simulink model "two_balloons_empirical"  (R2020b)
settings: Solver=VariableStepAuto  StartTime=0.0  StopTime=60*5  FixedStep=0.001  RelTol=1e-3
InitFcn:
  | seed1 = randi(100000);
  | seed2 = randi(200000);
model workspace (MAT data in the model file):
  dCoupling = 10
  kCoupling = 10
values from neighbouring files (symbols this model uses):
  bm = 2/1000    (= 0.002)    [optimiseB2.m]    (also in optimiseBO.m)
  Cd = a(4)    [comparisonPlot.m]    (also in optimiseB2.m = 0.185; optimiseBO.m = 0.185; params2.m = 0.185; sim_2balloon.m = 0.185)
  nH = x2nn.nH    [optimiseB2.m]    (also in optimiseBO.m = x.nH; params2.m = 10; sim_2balloon.m = x(2); sim_balloon.m = x(2))
  normalScaling = x2ll.normalScaling    [optimiseB2.m]    (also in optimiseBO.m = x.normalScaling; params2.m = 1; sim_2balloon.m = 0.259830816053; sim_balloon.m = x(5))
  nS = 1    [comparisonPlot.m]    (also in optimiseB2.m = x2nn.nS; optimiseBO.m = x.nS; params2.m = 0.025; sim_2balloon.m = x(3))
  nV = a(7)    [comparisonPlot.m]    (also in optimiseB2.m = x2nn.nV; optimiseBO.m = x.nV; params2.m = 0.5; sim_2balloon.m = x(1))
  rb = 0.16    [comparisonPlot.m]    (also in optimiseB2.m = 0.08; optimiseBO.m = 0.08; params2.m = 0.08; sim_2balloon.m = 0.08)
  rn = a(1)    [comparisonPlot.m]    (also in optimiseB2.m = 0.0625; optimiseBO.m = 0.0625; params2.m = 0.0625; sim_2balloon.m = 0.0625)
  seedX = randi(100000)    [optimiseB2.m]    (also in optimiseBO.m; params2.m; sim_2balloon.m; sim_balloon.m)
  seedX1 = randi(100000)    [optimiseB2.m]    (also in params2.m; sim_2balloon.m)
  seedY = randi(100000)    [optimiseB2.m]    (also in optimiseBO.m; params2.m; sim_2balloon.m; sim_balloon.m)
  seedY1 = randi(100000)    [optimiseB2.m]    (also in params2.m; sim_2balloon.m)
  seedZ = randi(100000)    [optimiseB2.m]    (also in optimiseBO.m; params2.m; sim_2balloon.m; sim_balloon.m)
  seedZ1 = randi(100000)    [optimiseB2.m]    (also in params2.m; sim_2balloon.m)
  theta = a(2)    [comparisonPlot.m]    (also in extract3D.m = deg2rad(-5); optimiseB2.m = x2ll.theta; optimiseBO.m = x.theta; params2.m = 3.5)
  V0 = a(3)    [comparisonPlot.m]    (also in optimiseB2.m = x2ll.V0; optimiseBO.m = x.V0; params2.m = 3.7; sim_2balloon.m = 1.01295922371)
undefined symbols (not defined in the file or in its folder): bm1
libraries: nesl_utility x19, sm_lib x10, eeGeneralControl x6
settings Model: Creator=toby  LastModifiedBy=BIRL

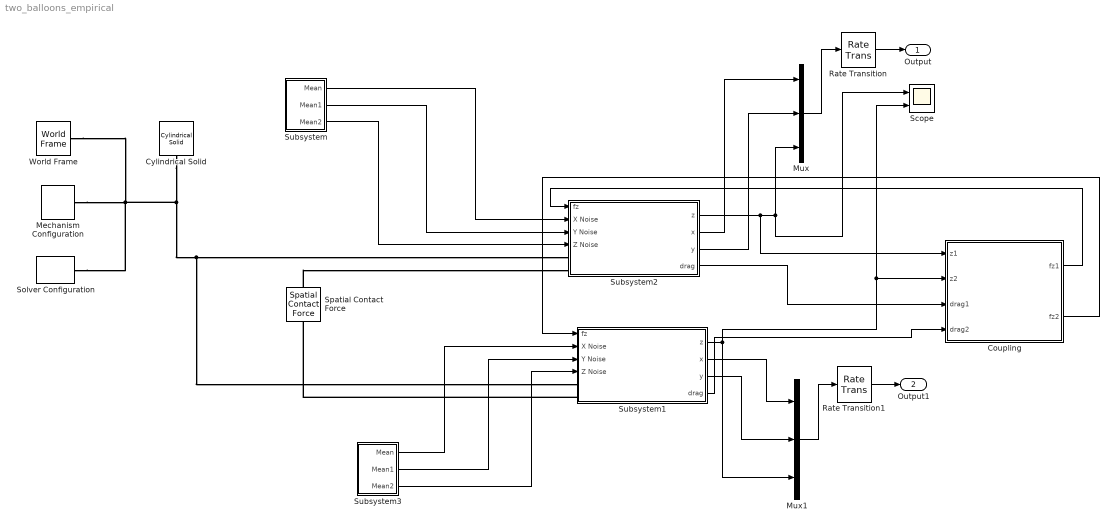
== system two_balloons_empirical ==
  Coupling : Subsystem
  Cylindrical Solid : sm_lib/Body Elements/Cylindrical Solid  GraphicAmbientColor=[0.15 0.15 0.15 1.0]  BasedOnType=Density  CenterOfMass=[0 0 0]  CenterOfMassUnits=m  GraphicDiffuseColor=[1.0 1.0 0.0]  CylinderLength=0.01  CylinderLengthUnits=m  CylinderRadius=rn  CylinderRadiusUnits=m  Density=1000  DensityUnits=kg/m^3  DoExposeReferenceFrame=on  GraphicEmissiveColor=[0.0 0.0 0.0 1.0]  ExportEntireGeometry=off  SerializedFrames=<Frames/>  MarkerShape=Sphere  MarkerSize=10  GraphicType=FromGeometry  InertiaType=CalculateFromGeometry  Mass=1  MassUnits=kg  MomentsOfInertia=[1 1 1]  MomentsOfInertiaUnits=kg*m^2  GraphicOpacity=1.0  ProductsOfInertia=[0 0 0]  ProductsOfInertiaUnits=kg*m^2  GraphicShininess=75  GraphicSpecularColor=[0.5 0.5 0.5 1.0]  GraphicVisPropType=SimpleVisualProperties
  Mechanism Configuration : sm_lib/Utilities/Mechanism Configuration  UniformGravity=Constant  GravityVector=[0 0 -9.81]  GravityVectorUnits=m/s^2  GravityUnits=m/s^2  LinearizationDelta=0.001  JointModeTransitionNonlinearIterations=2
  Mux : Mux  Inputs=3
  Mux1 : Mux  Inputs=3
  Rate Transition : RateTransition  OutPortSampleTime=1/40
  Rate Transition1 : RateTransition  OutPortSampleTime=1/40
  Scope : Scope  NumInputPorts=2
  Solver Configuration : nesl_utility/Solver Configuration  PhysicalDomain=network_engine_domain  SubClassName=solver  LeftPortType=input  RightPortType=generic  Tones=[]  Harmonics=[]  SimulateNoise=off  Profile=off  UseLocalSampling=off  EnableSwitchedLinearOptims=on  FrequencyDomain=off  UseCCode=off  RelTol=0.001  AbsTol=1e-06  MinStep=1e-09  ToWorkspace=off  RevertToSquareIcSolve=off  NumHomotopyIterations=100  PhasorMode=off  PhasorModeNumHarmonics=1  DoDC=off  ResidualTolerance=1e-9  UseLocalSolver=off  LocalSolverChoice=NE_BACKWARD_EULER_ADVANCER  LocalSolverSampleTime=.001  DoFixedCost=off  MaxNonlinIter=3  MaxModeIter=2  ComputeImpulses=off  ImpulseIterations=2  LinearAlgebra=Sparse  EquationFormulation=NE_TIME_EF  DelaysMemoryBudget=1024  AutomaticFiltering=on  FilteringTimeConstant=0.001  PartitionStorageMethod=AS_NEEDED  PartitionMemoryBudget=1024  PartitionMethod=FAST
  Spatial Contact Force : sm_lib/Forces and Torques/Spatial Contact Force  CoefficientOfDynamicFriction=0.1  CoefficientOfStaticFriction=0.1  NormalDamping=d  NormalDampingUnits=N/(m/s)  NormalStiffness=k  NormalStiffnessUnits=N/m  FrictionalCriticalVelocity=1e-3  FrictionalCriticalVelocityUnits=m/s  ZeroCrossDetectContactStartAndEnd=off  SenseFrictionalForceMagnitude=off  SenseNormalForceMagnitude=off  SenseSeparationDistance=off  NormalTransitionRegionWidth=tw  NormalTransitionRegionWidthUnits=m  FrictionType=SmoothStickSlip
  Subsystem : Subsystem
  Subsystem1 : Subsystem  mask{initialHeight=0.5, ix=0, iy=0, balloonRadius=80/1000, balloonMass=bm1}
      mask prompts: initialHeight "initial height"; balloonRadius "balloon radius"; balloonMass "balloon mass"
  Subsystem2 : Subsystem  mask{initialHeight=0.2, ix=0, iy=0, balloonRadius=80/1000, balloonMass=bm}
      mask prompts: initialHeight "initial height"; balloonRadius "balloon radius"; balloonMass "balloon mass"
  Subsystem3 : Subsystem
  World Frame : sm_lib/Frames and Transforms/World Frame
  Output : Outport
  Output1 : Outport  Port=2
  wires:
  Subsystem2/1(z) -> Coupling/1(z1), Scope/1, Mux/3
  Subsystem2/2(x) -> Mux/1
  Subsystem1/1(z) -> Scope/2, Coupling/2(z2), Mux1/3
  Subsystem1/2(x) -> Mux1/1
  Subsystem2/3(y) -> Mux/2
  Subsystem1/3(y) -> Mux1/2
  Rate Transition/1 -> Output/1
  Mux/1 -> Rate Transition/1
  Rate Transition1/1 -> Output1/1
  Mux1/1 -> Rate Transition1/1
  Coupling/1(fz1) -> Subsystem2/1(fz)
  Coupling/2(fz2) -> Subsystem1/1(fz)
  Subsystem2/4(drag) -> Coupling/3(drag1)
  Subsystem1/4(drag) -> Coupling/4(drag2)
  Subsystem/1(" Mean") -> Subsystem2/2(X Noise)
  Subsystem/2(" Mean1") -> Subsystem2/3(Y Noise)
  Subsystem/3(" Mean2") -> Subsystem2/4(Z Noise)
  Subsystem3/1(" Mean") -> Subsystem1/2(X Noise)
  Subsystem3/2(" Mean1") -> Subsystem1/3(Y Noise)
  Subsystem3/3(" Mean2") -> Subsystem1/4(Z Noise)
  connections:
  Solver Configuration/RConn1 -- Cylindrical Solid/RConn1 -- Subsystem1/LConn1 -- Subsystem2/LConn1 -- World Frame/RConn1 -- Mechanism Configuration/RConn1
  Spatial Contact Force/LConn1 -- Subsystem2/LConn2
  Subsystem1/LConn2 -- Spatial Contact Force/RConn1

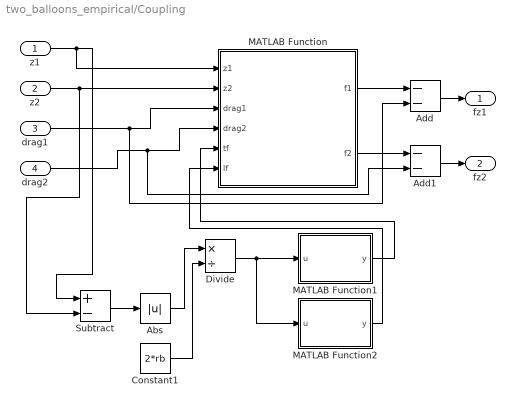
== system two_balloons_empirical/Coupling ==
  z1 : Inport
  z2 : Inport  Port=2
  drag1 : Inport  Port=3
  drag2 : Inport  Port=4
  Abs : Abs
  Add : Sum  Inputs=--
  Add1 : Sum  Inputs=--
  Constant1 : Constant  Value=2*rb
  Divide : Product  Inputs=*/
  MATLAB Function : MATLAB Function  TreatAsAtomicUnit=on
  MATLAB Function1 : MATLAB Function  TreatAsAtomicUnit=on
  MATLAB Function2 : MATLAB Function  TreatAsAtomicUnit=on
  Subtract : Sum  Inputs=+-
  fz1 : Outport
  fz2 : Outport  Port=2
  wires:
  drag1/1 -> Add/2, MATLAB Function/3(drag1)
  drag2/1 -> Add1/2, MATLAB Function/4(drag2)
  z1/1 -> MATLAB Function/1(z1), Subtract/1
  z2/1 -> Subtract/2, MATLAB Function/2(z2)
  Subtract/1 -> Abs/1
  Abs/1 -> Divide/1
  Constant1/1 -> Divide/2
  Divide/1 -> MATLAB Function2/1(u), MATLAB Function1/1(u)
  MATLAB Function1/1(y) -> MATLAB Function/5(tf)
  MATLAB Function2/1(y) -> MATLAB Function/6(lf)
  Add1/1 -> fz2/1
  Add/1 -> fz1/1
  MATLAB Function/1(f1) -> Add/1
  MATLAB Function/2(f2) -> Add1/1

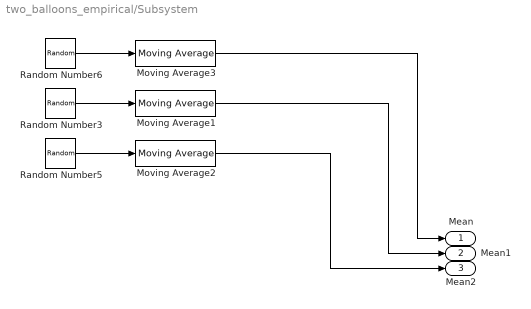
== system two_balloons_empirical/Subsystem ==
  Moving Average1 : eeGeneralControl/Moving Average  VariantControl=Variant1  LabelModeActiveChoice=Discrete  f=10  x0=0  Ts=nS/10
      settings: SourceProductBaseCode=PS
  Moving Average2 : eeGeneralControl/Moving Average  VariantControl=Variant1  LabelModeActiveChoice=Discrete  f=10  x0=0  Ts=nS/10
      settings: SourceProductBaseCode=PS
  Moving Average3 : eeGeneralControl/Moving Average  VariantControl=Variant1  LabelModeActiveChoice=Discrete  f=10  x0=0  Ts=nS/10
      settings: SourceProductBaseCode=PS
  Random Number3 : RandomNumber  Variance=nH  Seed=seedY  SampleTime=nS
  Random Number5 : RandomNumber  Variance=nV  Seed=seedZ  SampleTime=nS
  Random Number6 : RandomNumber  Variance=nH  Seed=seedX  SampleTime=nS
  " Mean" : Outport
  " Mean1" : Outport  Port=2
  " Mean2" : Outport  Port=3
  wires:
  Random Number3/1 -> Moving Average1/1
  Random Number5/1 -> Moving Average2/1
  Random Number6/1 -> Moving Average3/1
  Moving Average3/1 -> " Mean"/1
  Moving Average1/1 -> " Mean1"/1
  Moving Average2/1 -> " Mean2"/1

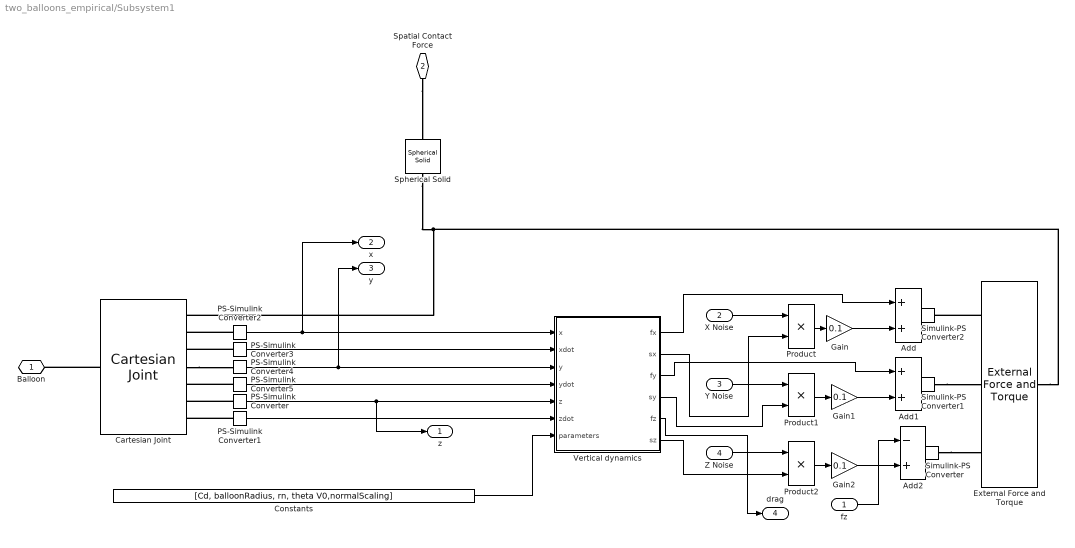
== system two_balloons_empirical/Subsystem1 ==
  fz : Inport
  X Noise : Inport  Port=2
  Y Noise : Inport  Port=3
  Z Noise : Inport  Port=4
  Add : Sum
  Add1 : Sum
  Add2 : Sum  Inputs=-+
  Cartesian Joint : sm_lib/Joints/Cartesian Joint  JointMode=Normal  SenseConstraintForce=off  SenseConstraintForceX=off  SenseConstraintForceY=off  SenseConstraintForceZ=off  SenseConstraintTorque=off  SenseConstraintTorqueX=off  SenseConstraintTorqueY=off  SenseConstraintTorqueZ=off  SenseTotalForce=off  SenseTotalForceX=off  SenseTotalForceY=off  SenseTotalForceZ=off  SenseTotalTorque=off  SenseTotalTorqueX=off  SenseTotalTorqueY=off  SenseTotalTorqueZ=off  CompositeWrenchDir=FollowerOnBase  CompositeWrenchFrame=BaseFrame  PxEquilibriumPosition=0  PxEquilibriumPositionUnits=m  PxSpringStiffness=0  PxSpringStiffnessUnits=N/m  PxDampingCoefficient=hd  PxDampingCoefficientUnits=N/(m/s)  PxTorqueActuationMode=NoTorque  PxMotionActuationMode=ComputedMotion  PxSensePosition=on  PxSenseVelocity=on  PxSenseAcceleration=off  PxSenseTorqueForce=off  PxSenseLowerLimitTorqueForce=off  PxSenseUpperLimitTorqueForce=off  PxLowerLimitSpecify=on  PxLowerLimitBound=-0.1  PxLowerLimitBoundUnits=m  PxLowerLimitStiffness=1e6  PxLowerLimitStiffnessUnits=N/m  PxLowerLimitDamping=1e3  PxLowerLimitDampingUnits=N/(m/s)  PxLowerLimitTransitionRegionWidth=1e-4  PxLowerLimitTransitionRegionWidthUnits=m  PxUpperLimitSpecify=on  PxUpperLimitBound=0.1  PxUpperLimitBoundUnits=m  PxUpperLimitStiffness=1e6  PxUpperLimitStiffnessUnits=N/m  PxUpperLimitDamping=1e3  PxUpperLimitDampingUnits=N/(m/s)  PxUpperLimitTransitionRegionWidth=1e-4  PxUpperLimitTransitionRegionWidthUnits=m  PxPositionTargetSpecify=on  PxPositionTargetPriority=High  PxPositionTargetValue=ix  PxPositionTargetValueUnits=m  PxVelocityTargetSpecify=off  PxVelocityTargetPriority=High  PxVelocityTargetValue=-0.75  PxVelocityTargetValueUnits=m/s  PyEquilibriumPosition=0  PyEquilibriumPositionUnits=m  PySpringStiffness=0  PySpringStiffnessUnits=N/m  PyDampingCoefficient=hd  PyDampingCoefficientUnits=N/(m/s)  PyTorqueActuationMode=NoTorque  PyMotionActuationMode=ComputedMotion  PySensePosition=on  PySenseVelocity=on  PySenseAcceleration=off  PySenseTorqueForce=off  PySenseLowerLimitTorqueForce=off  PySenseUpperLimitTorqueForce=off  PyLowerLimitSpecify=on  PyLowerLimitBound=-0.1  PyLowerLimitBoundUnits=m  PyLowerLimitStiffness=1e6  PyLowerLimitStiffnessUnits=N/m  PyLowerLimitDamping=1e3  PyLowerLimitDampingUnits=N/(m/s)  PyLowerLimitTransitionRegionWidth=1e-4  PyLowerLimitTransitionRegionWidthUnits=m  PyUpperLimitSpecify=on  PyUpperLimitBound=0.1  PyUpperLimitBoundUnits=m  PyUpperLimitStiffness=1e6  PyUpperLimitStiffnessUnits=N/m  PyUpperLimitDamping=1e3  PyUpperLimitDampingUnits=N/(m/s)  PyUpperLimitTransitionRegionWidth=1e-4  PyUpperLimitTransitionRegionWidthUnits=m  PyPositionTargetSpecify=on  PyPositionTargetPriority=High  PyPositionTargetValue=iy  PyPositionTargetValueUnits=m  PyVelocityTargetSpecify=off  PyVelocityTargetPriority=High  PyVelocityTargetValue=0  PyVelocityTargetValueUnits=m/s  PzEquilibriumPosition=0  PzEquilibriumPositionUnits=m  PzSpringStiffness=0  PzSpringStiffnessUnits=N/m  PzDampingCoefficient=0  PzDampingCoefficientUnits=N/(m/s)  PzTorqueActuationMode=NoTorque  PzMotionActuationMode=ComputedMotion  PzSensePosition=on  PzSenseVelocity=on  PzSenseAcceleration=off  PzSenseTorqueForce=off  PzSenseLowerLimitTorqueForce=off  PzSenseUpperLimitTorqueForce=off  PzLowerLimitSpecify=on  PzLowerLimitBound=0.1  PzLowerLimitBoundUnits=m  PzLowerLimitStiffness=1e6  PzLowerLimitStiffnessUnits=N/m  PzLowerLimitDamping=1e3  PzLowerLimitDampingUnits=N/(m/s)  PzLowerLimitTransitionRegionWidth=1e-4  PzLowerLimitTransitionRegionWidthUnits=m  PzUpperLimitSpecify=on  PzUpperLimitBound=1.7  PzUpperLimitBoundUnits=m  PzUpperLimitStiffness=1e6  PzUpperLimitStiffnessUnits=N/m  PzUpperLimitDamping=1e3  PzUpperLimitDampingUnits=N/(m/s)  PzUpperLimitTransitionRegionWidth=1e-4  PzUpperLimitTransitionRegionWidthUnits=m  PzPositionTargetSpecify=on  PzPositionTargetPriority=High  PzPositionTargetValue=initialHeight  PzPositionTargetValueUnits=m  PzVelocityTargetSpecify=off  PzVelocityTargetPriority=High  PzVelocityTargetValue=2.5  PzVelocityTargetValueUnits=m/s
  Constants : Constant  Value=[Cd, balloonRadius, rn, theta V0,normalScaling]
  External Force and Torque : sm_lib/Forces and Torques/External Force and Torque  ForceResolutionFrame=AttachedFrame  EnableForceX=on  EnableForceY=on  EnableForceZ=on  EnableForce=off  TorqueResolutionFrame=AttachedFrame  EnableTorqueX=off  EnableTorqueY=off  EnableTorqueZ=off  EnableTorque=off
  Gain : Gain  Gain=0.1
  Gain1 : Gain  Gain=0.1
  Gain2 : Gain  Gain=0.1
  PS-Simulink Converter{,1..5} (6 alike) : nesl_utility/PS-Simulink Converter  PhysicalDomain=network_engine_domain  SubClassName=ps_output  LeftPortType=input  RightPortType=output  PseudoPeriodic=off  Frequencies=[]  Unit=inherit  AffineConversion=off
  Product : Product
  Product1 : Product
  Product2 : Product
  Simulink-PS Converter : nesl_utility/Simulink-PS Converter  PhysicalDomain=network_engine_domain  SubClassName=ps_input  LeftPortType=input  RightPortType=output  PseudoPeriodic=off  Frequencies=[]  NoiseDistribution=none  NoiseParameters=[]  Unit=1  AffineConversion=off  FilteringAndDerivatives=provide  SimscapeFilterOrder=1  InputFilterTimeConstant=0.001  UdotUserProvided=0
  Simulink-PS Converter1 : nesl_utility/Simulink-PS Converter  PhysicalDomain=network_engine_domain  SubClassName=ps_input  LeftPortType=input  RightPortType=output  PseudoPeriodic=off  Frequencies=[]  NoiseDistribution=none  NoiseParameters=[]  Unit=1  AffineConversion=off  FilteringAndDerivatives=provide  SimscapeFilterOrder=1  InputFilterTimeConstant=0.001  UdotUserProvided=0
  Simulink-PS Converter2 : nesl_utility/Simulink-PS Converter  PhysicalDomain=network_engine_domain  SubClassName=ps_input  LeftPortType=input  RightPortType=output  PseudoPeriodic=off  Frequencies=[]  NoiseDistribution=none  NoiseParameters=[]  Unit=1  AffineConversion=off  FilteringAndDerivatives=provide  SimscapeFilterOrder=1  InputFilterTimeConstant=0.001  UdotUserProvided=0
  Spherical Solid : sm_lib/Body Elements/Spherical Solid  GraphicAmbientColor=[0.15 0.15 0.15 1.0]  BasedOnType=Mass  CenterOfMass=[0 0 0]  CenterOfMassUnits=m  GraphicDiffuseColor=[1.0 0.0 0.2]  Density=1000  DensityUnits=kg/m^3  DoExposeReferenceFrame=on  GraphicEmissiveColor=[0.0 0.0 0.0 1.0]  ExportEntireGeometry=on  SerializedExposedGeometries=<ExposedGeometries><ExposedGeometry><RawGeometryId>entire</RawGeometryId><ExposedGeometryId>G</ExposedGeometryId></ExposedGeometry></ExposedGeometries>  SerializedFrames=<Frames/>  MarkerShape=Sphere  MarkerSize=10  GraphicType=FromGeometry  InertiaType=CalculateFromGeometry  Mass=balloonMass  MassUnits=kg  MomentsOfInertia=[1 1 1]  MomentsOfInertiaUnits=kg*m^2  GraphicOpacity=1.0  ProductsOfInertia=[0 0 0]  ProductsOfInertiaUnits=kg*m^2  GraphicShininess=75  GraphicSpecularColor=[0.5 0.5 0.5 1.0]  SphereRadius=balloonRadius  SphereRadiusUnits=m  GraphicVisPropType=SimpleVisualProperties
  Vertical dynamics : MATLAB Function  TreatAsAtomicUnit=on
  Balloon : PMIOPort  Side=Left
  Spatial Contact Force : PMIOPort  Port=2  Side=Left
  z : Outport
  x : Outport  Port=2
  y : Outport  Port=3
  drag : Outport  Port=4
  wires:
  PS-Simulink Converter3/1 -> Vertical dynamics/2(xdot)
  PS-Simulink Converter5/1 -> Vertical dynamics/4(ydot)
  Constants/1 -> Vertical dynamics/7(parameters)
  PS-Simulink Converter1/1 -> Vertical dynamics/6(zdot)
  Vertical dynamics/6(sz) -> Product2/2
  X Noise/1 -> Product/1
  Vertical dynamics/4(sy) -> Product1/2
  Z Noise/1 -> Product2/1
  Y Noise/1 -> Product1/1
  Vertical dynamics/2(sx) -> Product/2
  Vertical dynamics/5(fz) -> drag/1
  Vertical dynamics/1(fx) -> Add/1
  Vertical dynamics/3(fy) -> Add1/1
  Add1/1 -> Simulink-PS Converter1/1
  Add/1 -> Simulink-PS Converter2/1
  Product/1 -> Gain/1
  Gain/1 -> Add/2
  Product1/1 -> Gain1/1
  Gain1/1 -> Add1/2
  Product2/1 -> Gain2/1
  Gain2/1 -> Add2/2
  Add2/1 -> Simulink-PS Converter/1
  fz/1 -> Add2/1
  PS-Simulink Converter2/1 -> Vertical dynamics/1(x), x/1
  PS-Simulink Converter4/1 -> Vertical dynamics/3(y), y/1
  PS-Simulink Converter/1 -> Vertical dynamics/5(z), z/1
  connections:
  PS-Simulink Converter/LConn1 -- Cartesian Joint/RConn6
  PS-Simulink Converter2/LConn1 -- Cartesian Joint/RConn2
  Spherical Solid/RConn1 -- External Force and Torque/RConn1 -- Cartesian Joint/RConn1
  Cartesian Joint/LConn1 -- Balloon/RConn1
  PS-Simulink Converter5/LConn1 -- Cartesian Joint/RConn5
  Cartesian Joint/RConn4 -- PS-Simulink Converter4/LConn1
  PS-Simulink Converter3/LConn1 -- Cartesian Joint/RConn3
  PS-Simulink Converter1/LConn1 -- Cartesian Joint/RConn7
  Spatial Contact Force/RConn1 -- Spherical Solid/LConn1
  External Force and Torque/LConn1 -- Simulink-PS Converter2/RConn1
  Simulink-PS Converter1/RConn1 -- External Force and Torque/LConn2
  Simulink-PS Converter/RConn1 -- External Force and Torque/LConn3

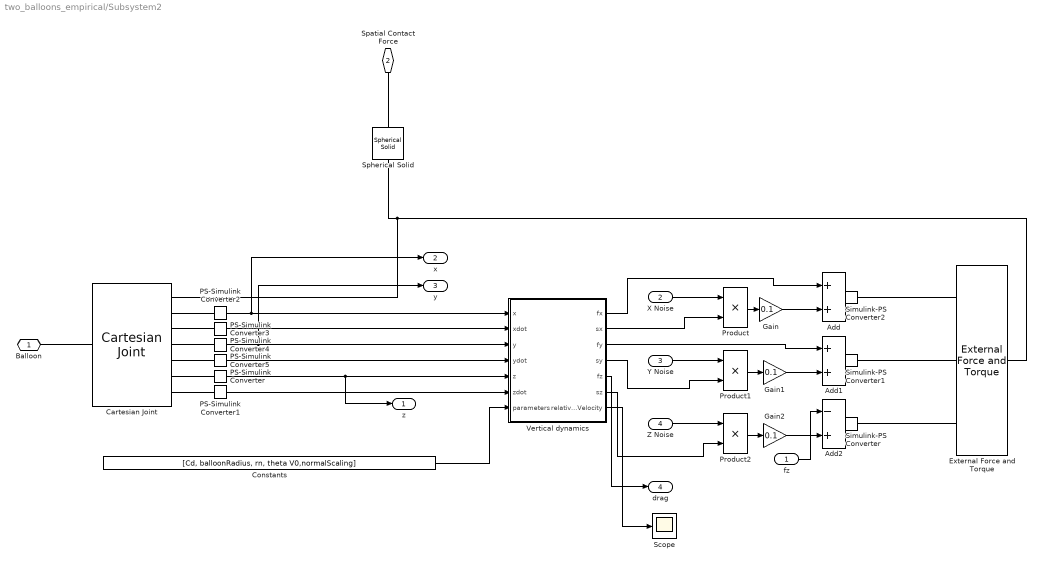
== system two_balloons_empirical/Subsystem2 ==
  fz : Inport
  X Noise : Inport  Port=2
  Y Noise : Inport  Port=3
  Z Noise : Inport  Port=4
  Add : Sum
  Add1 : Sum
  Add2 : Sum  Inputs=-+
  Cartesian Joint : sm_lib/Joints/Cartesian Joint  JointMode=Normal  SenseConstraintForce=off  SenseConstraintForceX=off  SenseConstraintForceY=off  SenseConstraintForceZ=off  SenseConstraintTorque=off  SenseConstraintTorqueX=off  SenseConstraintTorqueY=off  SenseConstraintTorqueZ=off  SenseTotalForce=off  SenseTotalForceX=off  SenseTotalForceY=off  SenseTotalForceZ=off  SenseTotalTorque=off  SenseTotalTorqueX=off  SenseTotalTorqueY=off  SenseTotalTorqueZ=off  CompositeWrenchDir=FollowerOnBase  CompositeWrenchFrame=BaseFrame  PxEquilibriumPosition=0  PxEquilibriumPositionUnits=m  PxSpringStiffness=0  PxSpringStiffnessUnits=N/m  PxDampingCoefficient=hd  PxDampingCoefficientUnits=N/(m/s)  PxTorqueActuationMode=NoTorque  PxMotionActuationMode=ComputedMotion  PxSensePosition=on  PxSenseVelocity=on  PxSenseAcceleration=off  PxSenseTorqueForce=off  PxSenseLowerLimitTorqueForce=off  PxSenseUpperLimitTorqueForce=off  PxLowerLimitSpecify=on  PxLowerLimitBound=-0.1  PxLowerLimitBoundUnits=m  PxLowerLimitStiffness=1e6  PxLowerLimitStiffnessUnits=N/m  PxLowerLimitDamping=1e3  PxLowerLimitDampingUnits=N/(m/s)  PxLowerLimitTransitionRegionWidth=1e-4  PxLowerLimitTransitionRegionWidthUnits=m  PxUpperLimitSpecify=on  PxUpperLimitBound=0.1  PxUpperLimitBoundUnits=m  PxUpperLimitStiffness=1e6  PxUpperLimitStiffnessUnits=N/m  PxUpperLimitDamping=1e3  PxUpperLimitDampingUnits=N/(m/s)  PxUpperLimitTransitionRegionWidth=1e-4  PxUpperLimitTransitionRegionWidthUnits=m  PxPositionTargetSpecify=on  PxPositionTargetPriority=High  PxPositionTargetValue=ix  PxPositionTargetValueUnits=m  PxVelocityTargetSpecify=off  PxVelocityTargetPriority=High  PxVelocityTargetValue=-0.75  PxVelocityTargetValueUnits=m/s  PyEquilibriumPosition=0  PyEquilibriumPositionUnits=m  PySpringStiffness=0  PySpringStiffnessUnits=N/m  PyDampingCoefficient=hd  PyDampingCoefficientUnits=N/(m/s)  PyTorqueActuationMode=NoTorque  PyMotionActuationMode=ComputedMotion  PySensePosition=on  PySenseVelocity=on  PySenseAcceleration=off  PySenseTorqueForce=off  PySenseLowerLimitTorqueForce=off  PySenseUpperLimitTorqueForce=off  PyLowerLimitSpecify=on  PyLowerLimitBound=-0.1  PyLowerLimitBoundUnits=m  PyLowerLimitStiffness=1e6  PyLowerLimitStiffnessUnits=N/m  PyLowerLimitDamping=1e3  PyLowerLimitDampingUnits=N/(m/s)  PyLowerLimitTransitionRegionWidth=1e-4  PyLowerLimitTransitionRegionWidthUnits=m  PyUpperLimitSpecify=on  PyUpperLimitBound=0.1  PyUpperLimitBoundUnits=m  PyUpperLimitStiffness=1e6  PyUpperLimitStiffnessUnits=N/m  PyUpperLimitDamping=1e3  PyUpperLimitDampingUnits=N/(m/s)  PyUpperLimitTransitionRegionWidth=1e-4  PyUpperLimitTransitionRegionWidthUnits=m  PyPositionTargetSpecify=on  PyPositionTargetPriority=High  PyPositionTargetValue=iy  PyPositionTargetValueUnits=m  PyVelocityTargetSpecify=off  PyVelocityTargetPriority=High  PyVelocityTargetValue=0  PyVelocityTargetValueUnits=m/s  PzEquilibriumPosition=0  PzEquilibriumPositionUnits=m  PzSpringStiffness=0  PzSpringStiffnessUnits=N/m  PzDampingCoefficient=0  PzDampingCoefficientUnits=N/(m/s)  PzTorqueActuationMode=NoTorque  PzMotionActuationMode=ComputedMotion  PzSensePosition=on  PzSenseVelocity=on  PzSenseAcceleration=off  PzSenseTorqueForce=off  PzSenseLowerLimitTorqueForce=off  PzSenseUpperLimitTorqueForce=off  PzLowerLimitSpecify=on  PzLowerLimitBound=0.1  PzLowerLimitBoundUnits=m  PzLowerLimitStiffness=1e6  PzLowerLimitStiffnessUnits=N/m  PzLowerLimitDamping=1e3  PzLowerLimitDampingUnits=N/(m/s)  PzLowerLimitTransitionRegionWidth=1e-4  PzLowerLimitTransitionRegionWidthUnits=m  PzUpperLimitSpecify=on  PzUpperLimitBound=1.7  PzUpperLimitBoundUnits=m  PzUpperLimitStiffness=1e6  PzUpperLimitStiffnessUnits=N/m  PzUpperLimitDamping=1e3  PzUpperLimitDampingUnits=N/(m/s)  PzUpperLimitTransitionRegionWidth=1e-4  PzUpperLimitTransitionRegionWidthUnits=m  PzPositionTargetSpecify=on  PzPositionTargetPriority=High  PzPositionTargetValue=initialHeight  PzPositionTargetValueUnits=m  PzVelocityTargetSpecify=off  PzVelocityTargetPriority=High  PzVelocityTargetValue=2.5  PzVelocityTargetValueUnits=m/s
  Constants : Constant  Value=[Cd, balloonRadius, rn, theta V0,normalScaling]
  External Force and Torque : sm_lib/Forces and Torques/External Force and Torque  ForceResolutionFrame=AttachedFrame  EnableForceX=on  EnableForceY=on  EnableForceZ=on  EnableForce=off  TorqueResolutionFrame=AttachedFrame  EnableTorqueX=off  EnableTorqueY=off  EnableTorqueZ=off  EnableTorque=off
  Gain : Gain  Gain=0.1
  Gain1 : Gain  Gain=0.1
  Gain2 : Gain  Gain=0.1
  PS-Simulink Converter{,1..5} (6 alike) : nesl_utility/PS-Simulink Converter  PhysicalDomain=network_engine_domain  SubClassName=ps_output  LeftPortType=input  RightPortType=output  PseudoPeriodic=off  Frequencies=[]  Unit=inherit  AffineConversion=off
  Product : Product
  Product1 : Product
  Product2 : Product
  Scope : Scope
  Simulink-PS Converter : nesl_utility/Simulink-PS Converter  PhysicalDomain=network_engine_domain  SubClassName=ps_input  LeftPortType=input  RightPortType=output  PseudoPeriodic=off  Frequencies=[]  NoiseDistribution=none  NoiseParameters=[]  Unit=1  AffineConversion=off  FilteringAndDerivatives=provide  SimscapeFilterOrder=1  InputFilterTimeConstant=0.001  UdotUserProvided=0
  Simulink-PS Converter1 : nesl_utility/Simulink-PS Converter  PhysicalDomain=network_engine_domain  SubClassName=ps_input  LeftPortType=input  RightPortType=output  PseudoPeriodic=off  Frequencies=[]  NoiseDistribution=none  NoiseParameters=[]  Unit=1  AffineConversion=off  FilteringAndDerivatives=provide  SimscapeFilterOrder=1  InputFilterTimeConstant=0.001  UdotUserProvided=0
  Simulink-PS Converter2 : nesl_utility/Simulink-PS Converter  PhysicalDomain=network_engine_domain  SubClassName=ps_input  LeftPortType=input  RightPortType=output  PseudoPeriodic=off  Frequencies=[]  NoiseDistribution=none  NoiseParameters=[]  Unit=1  AffineConversion=off  FilteringAndDerivatives=provide  SimscapeFilterOrder=1  InputFilterTimeConstant=0.001  UdotUserProvided=0
  Spherical Solid : sm_lib/Body Elements/Spherical Solid  GraphicAmbientColor=[0.15 0.15 0.15 1.0]  BasedOnType=Mass  CenterOfMass=[0 0 0]  CenterOfMassUnits=m  GraphicDiffuseColor=[0.0 0.0 1.0]  Density=1000  DensityUnits=kg/m^3  DoExposeReferenceFrame=on  GraphicEmissiveColor=[0.0 0.0 0.0 1.0]  ExportEntireGeometry=on  SerializedExposedGeometries=<ExposedGeometries><ExposedGeometry><RawGeometryId>entire</RawGeometryId><ExposedGeometryId>G</ExposedGeometryId></ExposedGeometry></ExposedGeometries>  SerializedFrames=<Frames/>  MarkerShape=Sphere  MarkerSize=10  GraphicType=FromGeometry  InertiaType=CalculateFromGeometry  Mass=balloonMass  MassUnits=kg  MomentsOfInertia=[1 1 1]  MomentsOfInertiaUnits=kg*m^2  GraphicOpacity=1.0  ProductsOfInertia=[0 0 0]  ProductsOfInertiaUnits=kg*m^2  GraphicShininess=75  GraphicSpecularColor=[0.5 0.5 0.5 1.0]  SphereRadius=balloonRadius  SphereRadiusUnits=m  GraphicVisPropType=SimpleVisualProperties
  Vertical dynamics : MATLAB Function  TreatAsAtomicUnit=on
  Balloon : PMIOPort  Side=Left
  Spatial Contact Force : PMIOPort  Port=2  Side=Left
  z : Outport
  x : Outport  Port=2
  y : Outport  Port=3
  drag : Outport  Port=4
  wires:
  PS-Simulink Converter3/1 -> Vertical dynamics/2(xdot)
  PS-Simulink Converter5/1 -> Vertical dynamics/4(ydot)
  Constants/1 -> Vertical dynamics/7(parameters)
  Vertical dynamics/6(sz) -> Product2/2
  X Noise/1 -> Product/1
  Vertical dynamics/4(sy) -> Product1/2
  Z Noise/1 -> Product2/1
  Y Noise/1 -> Product1/1
  Vertical dynamics/2(sx) -> Product/2
  Vertical dynamics/5(fz) -> drag/1
  Vertical dynamics/1(fx) -> Add/1
  Vertical dynamics/3(fy) -> Add1/1
  Add2/1 -> Simulink-PS Converter/1
  Add1/1 -> Simulink-PS Converter1/1
  Add/1 -> Simulink-PS Converter2/1
  Gain/1 -> Add/2
  Product/1 -> Gain/1
  Product1/1 -> Gain1/1
  Gain1/1 -> Add1/2
  Gain2/1 -> Add2/2
  Product2/1 -> Gain2/1
  PS-Simulink Converter1/1 -> Vertical dynamics/6(zdot)
  PS-Simulink Converter/1 -> Vertical dynamics/5(z), z/1
  Vertical dynamics/7(relativeVelocity) -> Scope/1
  fz/1 -> Add2/1
  PS-Simulink Converter2/1 -> x/1, Vertical dynamics/1(x)
  PS-Simulink Converter4/1 -> y/1, Vertical dynamics/3(y)
  connections:
  PS-Simulink Converter/LConn1 -- Cartesian Joint/RConn6
  PS-Simulink Converter2/LConn1 -- Cartesian Joint/RConn2
  Spherical Solid/RConn1 -- Cartesian Joint/RConn1 -- External Force and Torque/RConn1
  Cartesian Joint/LConn1 -- Balloon/RConn1
  PS-Simulink Converter5/LConn1 -- Cartesian Joint/RConn5
  Cartesian Joint/RConn4 -- PS-Simulink Converter4/LConn1
  PS-Simulink Converter3/LConn1 -- Cartesian Joint/RConn3
  PS-Simulink Converter1/LConn1 -- Cartesian Joint/RConn7
  Spatial Contact Force/RConn1 -- Spherical Solid/LConn1
  External Force and Torque/LConn1 -- Simulink-PS Converter2/RConn1
  Simulink-PS Converter1/RConn1 -- External Force and Torque/LConn2
  Simulink-PS Converter/RConn1 -- External Force and Torque/LConn3

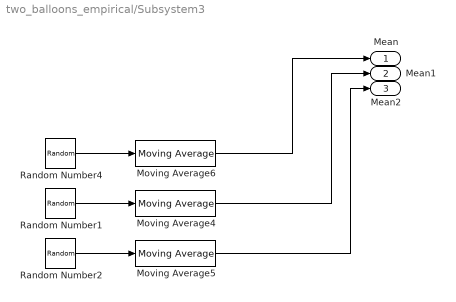
== system two_balloons_empirical/Subsystem3 ==
  Moving Average4 : eeGeneralControl/Moving Average  VariantControl=Variant1  LabelModeActiveChoice=Discrete  f=10  x0=0  Ts=nS/10
      settings: SourceProductBaseCode=PS
  Moving Average5 : eeGeneralControl/Moving Average  VariantControl=Variant1  LabelModeActiveChoice=Discrete  f=10  x0=0  Ts=nS/10
      settings: SourceProductBaseCode=PS
  Moving Average6 : eeGeneralControl/Moving Average  VariantControl=Variant1  LabelModeActiveChoice=Discrete  f=10  x0=0  Ts=nS/10
      settings: SourceProductBaseCode=PS
  Random Number1 : RandomNumber  Variance=nH  Seed=seedY1  SampleTime=nS
  Random Number2 : RandomNumber  Variance=nV  Seed=seedZ1  SampleTime=nS
  Random Number4 : RandomNumber  Variance=nH  Seed=seedX1  SampleTime=nS
  " Mean" : Outport
  " Mean1" : Outport  Port=2
  " Mean2" : Outport  Port=3
  wires:
  Random Number1/1 -> Moving Average4/1
  Random Number2/1 -> Moving Average5/1
  Moving Average5/1 -> " Mean2"/1
  Random Number4/1 -> Moving Average6/1
  Moving Average6/1 -> " Mean"/1
  Moving Average4/1 -> " Mean1"/1

== matlab function two_balloons_empirical/Coupling/MATLAB Function1 ==
  data: u input; y output
function y = trailingFit(u)

y = u;

== matlab function two_balloons_empirical/Coupling/MATLAB Function ==
  data: z1 input; f1 output; z2 input; drag1 input; drag2 input; f2 output; tf input; lf input
function [f1,f2] = fcn(z1,z2, drag1, drag2, tf, lf)

    R = abs(z1-z2);
    D = 0.16;

    if R/D < 4.5;
        rT = tf;
        rL = lf;
    else;
        rT = 1;
        rL = 1;
    end

    if z1<z2;
        f1 = rL*drag1;
        f2 = rT*drag2;
    else;
        f2 = rL*drag2;
        f1 = rT*drag1;
    end


end

== matlab function two_balloons_empirical/Subsystem2/Vertical dynamics ==
  data: fx output; sx output; fy output; sy output; x input; xdot input; y input; ydot input; z input; fz output; zdot input; parameters input; sz output; relativeVelocity output
function [fx,sx,fy,sy,fz,sz, relativeVelocity] = fcn(x,xdot,y,ydot,z,zdot,parameters)

Cd = parameters(1);
rb = parameters(2);
rn = parameters(3);
theta = deg2rad(parameters(4)); 
V0 = parameters(5); 
normalScaling = parameters(6); 

%% Vertical forces

%Horizontal plane displacement
[rotation, rDisplacement] = cart2pol(x,y);

%flow radius
rFlow = rn+z*tan(theta);

%Peak flow velocity
meanFlowVelocity = V0*rn^2/(rFlow)^2;

%Velocity under ball
vFlowActual = flowSpeed(meanFlowVelocity,normalScaling*rFlow,rDisplacement);

%Relative
relativeVelocity = vFlowActual - zdot;

reZ = (1.22 * abs(relativeVelocity) * 2*rb)/(1.81*10^-5);

%Force
fz = sign(rFlow) * 0.5 * Cd * (pi * rb^2) * 1.22 * relativeVelocity^2;

%% Horizontal X forces

innerR = abs(x)-rb;
outerR = abs(x)+rb;
vInner = flowSpeed(meanFlowVelocity,normalScaling*rFlow,innerR);
vOuter = flowSpeed(meanFlowVelocity,normalScaling*rFlow,outerR);
fx = 0.5*1.22*(vOuter^2-vInner^2)*sign(x);

%% Horizontal Y forces
innerR = abs(y)-rb;%3*rb/8;
outerR = abs(y)+rb;%3*rb/8;
vInner = flowSpeed(meanFlowVelocity,normalScaling*rFlow,innerR);
vOuter = flowSpeed(meanFlowVelocity,normalScaling*rFlow,outerR);
fy = 0.5*1.22*(vOuter^2-vInner^2)*sign(y);

%% Drag
dragX = 0.5 * Cd * pi * rb^2 * 1.22 * xdot;
fx = fx - dragX;

dragY = 0.5 * Cd * pi * rb^2 * 1.22 * ydot;
fy = fy - dragY;

%% Force scalings
sx = flowSpeed(meanFlowVelocity,normalScaling*rFlow,x)/flowSpeed(meanFlowVelocity,rFlow,0);
sy = flowSpeed(meanFlowVelocity,normalScaling*rFlow,y)/flowSpeed(meanFlowVelocity,rFlow,0);
sz = flowSpeed(meanFlowVelocity,normalScaling*rFlow,rDisplacement)/flowSpeed(meanFlowVelocity,rFlow,0);

== matlab function two_balloons_empirical/Subsystem1/Vertical dynamics ==
  data: fx output; sx output; fy output; sy output; x input; xdot input; y input; ydot input; z input; fz output; zdot input; parameters input; sz output

function [fx,sx,fy,sy,fz,sz] = fcn(x,xdot,y,ydot,z,zdot,parameters)

Cd = parameters(1);
rb = parameters(2);
rn = parameters(3);
theta = deg2rad(parameters(4)); 
V0 = parameters(5); 
normalScaling = parameters(6); 

%% Vertical forces

%Horizontal plane displacement
[rotation, rDisplacement] = cart2pol(x,y);

%flow radius
rFlow = rn+z*tan(theta);

%Peak flow velocity
meanFlowVelocity = V0*rn^2/(rFlow)^2;

%Velocity under ball
vFlowActual = flowSpeed(meanFlowVelocity,normalScaling*rFlow,rDisplacement);

%Relative
relativeVelocity = vFlowActual - zdot;

reZ = (1.22 * abs(relativeVelocity) * 2*rb)/(1.81*10^-5);

%Force
fz = sign(rFlow) * 0.5 * Cd * (pi * rb^2) * 1.22 * relativeVelocity^2;

%% Horizontal X forces

innerR = abs(x)-rb;
outerR = abs(x)+rb;
vInner = flowSpeed(meanFlowVelocity,normalScaling*rFlow,innerR);
vOuter = flowSpeed(meanFlowVelocity,normalScaling*rFlow,outerR);
fx = 0.5*1.22*(vOuter^2-vInner^2)*sign(x);

%% Horizontal Y forces
innerR = abs(y)-rb;%3*rb/8;
outerR = abs(y)+rb;%3*rb/8;
vInner = flowSpeed(meanFlowVelocity,normalScaling*rFlow,innerR);
vOuter = flowSpeed(meanFlowVelocity,normalScaling*rFlow,outerR);
fy = 0.5*1.22*(vOuter^2-vInner^2)*sign(y);

%% Drag
dragX = 0.5 * Cd * pi * rb^2 * 1.22 * xdot;
fx = fx - dragX;

dragY = 0.5 * Cd * pi * rb^2 * 1.22 * ydot;
fy = fy - dragY;

%% Force scalings
sx = flowSpeed(meanFlowVelocity,normalScaling*rFlow,x)/flowSpeed(meanFlowVelocity,rFlow,0);
sy = flowSpeed(meanFlowVelocity,normalScaling*rFlow,y)/flowSpeed(meanFlowVelocity,rFlow,0);
sz = flowSpeed(meanFlowVelocity,normalScaling*rFlow,rDisplacement)/flowSpeed(meanFlowVelocity,rFlow,0);

== matlab function two_balloons_empirical/Coupling/MATLAB Function2 ==
  data: u input; y output
function y = leadingFit(u)

y = u;
